simulink model "ExampleUniformVar"  (R2017b)
settings: Solver=VariableStepAuto  StartTime=0.0  StopTime=1000000000000000000.0  RelTol=1e-3
undefined symbols (not defined in the file or in its folder): add
settings Model: Creator=aarrieta  LastModifiedBy=aarrieta

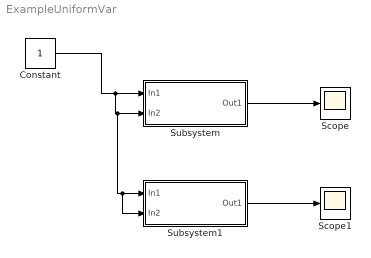
== system ExampleUniformVar ==
  Constant : Constant
  Scope : Scope
  Scope1 : Scope
  Subsystem : Subsystem
  Subsystem1 : Subsystem
  wires:
  Constant/1 -> Subsystem1/2(In2), Subsystem1/1(In1), Subsystem/2(In2), Subsystem/1(In1)
  Subsystem/1(Out1) -> Scope/1
  Subsystem1/1(Out1) -> Scope1/1

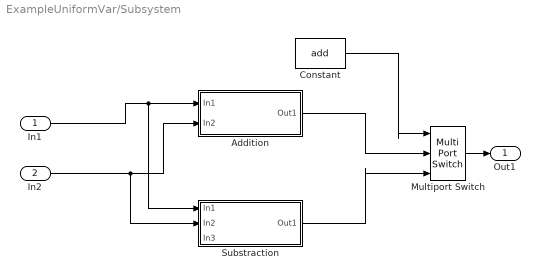
== system ExampleUniformVar/Subsystem ==
  In1 : Inport
  In2 : Inport  Port=2
  Addition : Subsystem
  Constant : Constant  Value=add
  Multiport Switch : MultiPortSwitch  Inputs=2
  Substraction : Subsystem
  Out1 : Outport
  wires:
  In1/1 -> Substraction/1(In1), Addition/1(In1)
  In2/1 -> Substraction/2(In2), Addition/2(In2)
  Substraction/1(Out1) -> Multiport Switch/3
  Addition/1(Out1) -> Multiport Switch/2
  Constant/1 -> Multiport Switch/1
  Multiport Switch/1 -> Out1/1

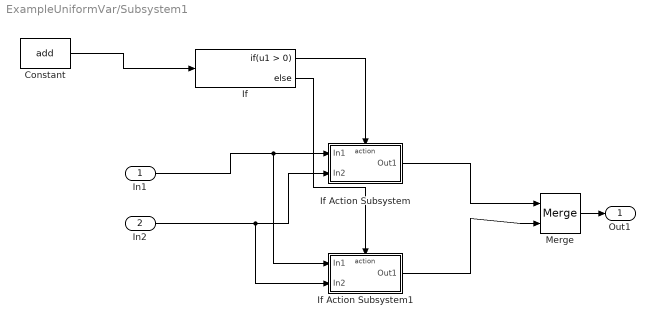
== system ExampleUniformVar/Subsystem1 ==
  In1 : Inport
  In2 : Inport  Port=2
  Constant : Constant  Value=add
  If : If
  If Action Subsystem : Subsystem  TreatAsAtomicUnit=on
  If Action Subsystem1 : Subsystem  TreatAsAtomicUnit=on
  Merge : Merge
  Out1 : Outport
  wires:
  Constant/1 -> If/1
  If Action Subsystem/1(Out1) -> Merge/1
  If Action Subsystem1/1(Out1) -> Merge/2
  In2/1 -> If Action Subsystem1/2(In2), If Action Subsystem/2(In2)
  In1/1 -> If Action Subsystem1/1(In1), If Action Subsystem/1(In1)
  Merge/1 -> Out1/1
  If/1 -> If Action Subsystem/Action
  If/2 -> If Action Subsystem1/Action

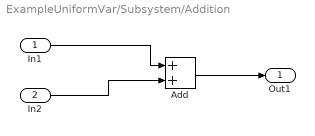
== system ExampleUniformVar/Subsystem/Addition ==
  In1 : Inport
  In2 : Inport  Port=2
  Add : Sum
  Out1 : Outport
  wires:
  In1/1 -> Add/1
  In2/1 -> Add/2
  Add/1 -> Out1/1

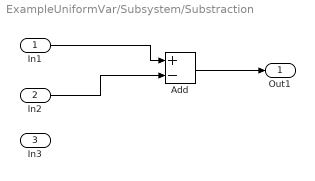
== system ExampleUniformVar/Subsystem/Substraction ==
  In1 : Inport
  In2 : Inport  Port=2
  In3 : Inport  Port=3
  Add : Sum  Inputs=+-
  Out1 : Outport
  wires:
  In1/1 -> Add/1
  In2/1 -> Add/2
  Add/1 -> Out1/1

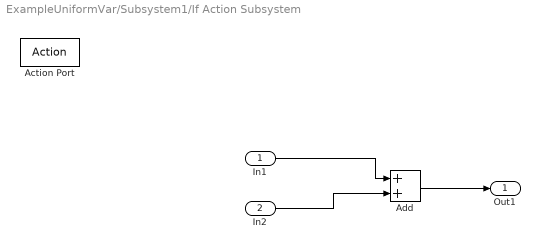
== system ExampleUniformVar/Subsystem1/If Action Subsystem ==
  In1 : Inport
  In2 : Inport  Port=2
  Action Port : ActionPort  ActionType=then
  Add : Sum
  Out1 : Outport
  wires:
  In2/1 -> Add/2
  Add/1 -> Out1/1
  In1/1 -> Add/1

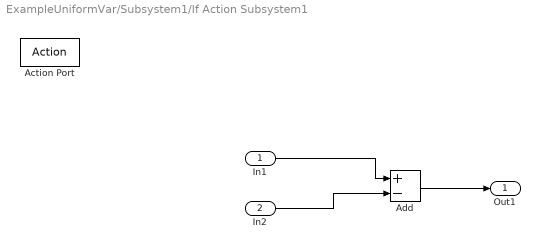
== system ExampleUniformVar/Subsystem1/If Action Subsystem1 ==
  In1 : Inport
  In2 : Inport  Port=2
  Action Port : ActionPort  ActionType=else
  Add : Sum  Inputs=+-
  Out1 : Outport
  wires:
  In1/1 -> Add/1
  Add/1 -> Out1/1
  In2/1 -> Add/2
